simulink model "PSS2B_block"  (R2020a)
settings: Solver=FixedStepAuto  StartTime=0.0  StopTime=16.5  FixedStep=0.005  RelTol=1e-3
undefined symbols (not defined in the file): K_S1, K_S2, K_S3, T_1, T_10, T_11, T_2, T_3, T_4, T_6, T_7, T_8, T_9, T_w1, T_w2, T_w3, T_w4, V_S1MAX, V_S1MIN, V_S2MAX, V_S2MIN, V_STMAX, V_STMIN
settings Model: Creator=meagh  LastModifiedBy=meagh

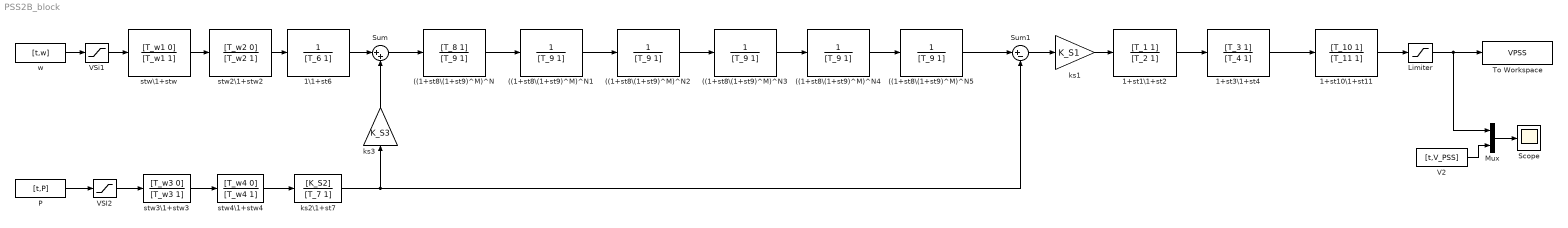
== system PSS2B_block ==
  ((1+st8\(1+st9)^M)^N : TransferFcn  Numerator=[T_8 1]  Denominator=[T_9 1]
  ((1+st8\(1+st9)^M)^N{1..5} (5 alike) : TransferFcn  Denominator=[T_9 1]
  1+st10\1+st11 : TransferFcn  Numerator=[T_10 1]  Denominator=[T_11 1]
  1+st1\1+st2 : TransferFcn  Numerator=[T_1 1]  Denominator=[T_2 1]
  1+st3\1+st4 : TransferFcn  Numerator=[T_3 1]  Denominator=[T_4 1]
  1\1+st6 : TransferFcn  Denominator=[T_6 1]
  "Limiter " : Saturate  UpperLimit=V_STMAX  LowerLimit=V_STMIN
  Mux : Mux  Inputs=2
  P : FromWorkspace  VariableName=[t,P]
  Scope : Scope
  Sum : Sum  Inputs=|++
  Sum1 : Sum  Inputs=|+-
  To Workspace : ToWorkspace  VariableName=VPSS  SaveFormat=Timeseries  SampleTime=-1
  V2 : FromWorkspace  VariableName=[t,V_PSS]
  VSI2 : Saturate  UpperLimit=V_S2MAX  LowerLimit=V_S2MIN
  VSi1 : Saturate  UpperLimit=V_S1MAX  LowerLimit=V_S1MIN
  ks1 : Gain  Gain=K_S1  SaturateOnIntegerOverflow=on  OutDataTypeStr=Inherit: Same as input  ParamDataTypeStr=Inherit: Same as input
  ks2\1+st7 : TransferFcn  Numerator=[K_S2]  Denominator=[T_7 1]
  ks3 : Gain  Gain=K_S3  SaturateOnIntegerOverflow=on  OutDataTypeStr=Inherit: Same as input  ParamDataTypeStr=Inherit: Same as input
  stw2\1+stw2 : TransferFcn  Numerator=[T_w2 0]  Denominator=[T_w2 1]
  stw3\1+stw3 : TransferFcn  Numerator=[T_w3 0]  Denominator=[T_w3 1]
  stw4\1+stw4 : TransferFcn  Numerator=[T_w4 0]  Denominator=[T_w4 1]
  stw\1+stw : TransferFcn  Numerator=[T_w1 0]  Denominator=[T_w1 1]
  w : FromWorkspace  VariableName=[t,w]
  wires:
  ks1/1 -> 1+st1\1+st2/1
  1+st3\1+st4/1 -> 1+st10\1+st11/1
  stw3\1+stw3/1 -> stw4\1+stw4/1
  ks2\1+st7/1 -> Sum1/2, ks3/1
  stw2\1+stw2/1 -> 1\1+st6/1
  ks3/1 -> Sum/2
  ((1+st8\(1+st9)^M)^N/1 -> ((1+st8\(1+st9)^M)^N1/1
  Sum1/1 -> ks1/1
  Sum/1 -> ((1+st8\(1+st9)^M)^N/1
  stw4\1+stw4/1 -> ks2\1+st7/1
  1\1+st6/1 -> Sum/1
  stw\1+stw/1 -> stw2\1+stw2/1
  1+st1\1+st2/1 -> 1+st3\1+st4/1
  P/1 -> VSI2/1
  VSI2/1 -> stw3\1+stw3/1
  VSi1/1 -> stw\1+stw/1
  w/1 -> VSi1/1
  1+st10\1+st11/1 -> "Limiter "/1
  V2/1 -> Mux/2
  "Limiter "/1 -> Mux/1, To Workspace/1
  Mux/1 -> Scope/1
  ((1+st8\(1+st9)^M)^N1/1 -> ((1+st8\(1+st9)^M)^N2/1
  ((1+st8\(1+st9)^M)^N2/1 -> ((1+st8\(1+st9)^M)^N3/1
  ((1+st8\(1+st9)^M)^N3/1 -> ((1+st8\(1+st9)^M)^N4/1
  ((1+st8\(1+st9)^M)^N4/1 -> ((1+st8\(1+st9)^M)^N5/1
  ((1+st8\(1+st9)^M)^N5/1 -> Sum1/1
